simulink model "L22B3"  (R2015a)
settings: Solver=ode45  StartTime=0.0  StopTime=1  MaxStep=0.001  RelTol=1e-3
values from neighbouring files (symbols this model uses):
  bB3 = 1138537    [L22m.m]
  c = 10000    [L22m.m]
  fi1 = -294.11    [L22m.m]
  fi2 = -10740    [L22m.m]
  J = 0.71e-3    (= 0.00071)    [L22m.m]
  kB3 = 5*1e+7    (= 50000000)    [L22m.m]
  ke = 0.33    [L22m.m]
  km = ke    (= 0.33)    [L22m.m]
  kp = 35    [L22m.m]
  La = 14.28e-3    (= 0.01428)    [L22m.m]
  Ra = 4.2    [L22m.m]
  v = -12    [L22m.m]
  vTime = 0.6    [L22m.m]
  w = 20    [L22m.m]
settings Model: Creator=B014-5  LastModifiedBy=B014-5

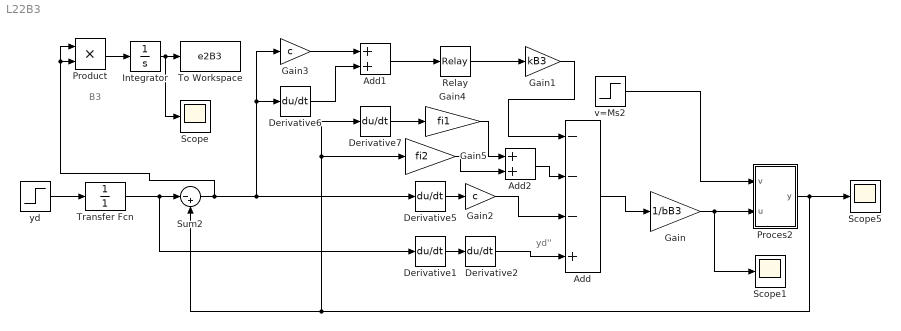
== system L22B3 ==
  note: yd''
  note: B3
  Add : Sum  Inputs=---+
  Add1 : Sum
  Add2 : Sum
  Derivative{1..2,5..7} (5 alike) : Derivative  CoefficientInTFapproximation=1e+5
  Gain : Gain  Gain=1/bB3
  Gain1 : Gain  Gain=kB3
  Gain2 : Gain  Gain=c
  Gain3 : Gain  Gain=c
  Gain4 : Gain  Gain=fi1
  Gain5 : Gain  Gain=fi2
  Integrator : Integrator
  Proces2 : Subsystem
  Product : Product
  Relay : Relay  OnSwitchValue=0  OffSwitchValue=0  OffOutputValue=-1  ZeroCross=off
  Scope : Scope
  Scope1 : Scope
      settings: YMin=-4.25e+105  YMax=0
  Scope5 : Scope
      settings: YMin=-4.25e+105  YMax=0  SaveName=ScopeData6
  Sum2 : Sum  Inputs=|-+
  To Workspace : ToWorkspace  VariableName=e2B3  SampleTime=-1
  Transfer Fcn : TransferFcn  Denominator=[0.0 1]
  v=Ms2 : Step  Time=vTime  After=v  SampleTime=0
  yd : Step  Time=0  After=w  SampleTime=0
  wires:
  Derivative1/1 -> Derivative2/1
  Proces2/1(y) -> Scope5/1, Sum2/2, Gain5/1, Derivative7/1
  Derivative5/1 -> Gain2/1
  v=Ms2/1 -> Proces2/1(v)
  Add/1 -> Gain/1
  Gain2/1 -> Add/3
  Add1/1 -> Relay/1
  Derivative6/1 -> Add1/2
  Gain3/1 -> Add1/1
  Relay/1 -> Gain1/1
  Gain1/1 -> Add/1
  Derivative7/1 -> Gain4/1
  Gain/1 -> Scope1/1, Proces2/2(u)
  Sum2/1 -> Gain3/1, Derivative6/1, Derivative5/1, Product/1, Product/2
  Product/1 -> Integrator/1
  Integrator/1 -> Scope/1, To Workspace/1
  Derivative2/1 -> Add/4
  Add2/1 -> Add/2
  Gain4/1 -> Add2/1
  Gain5/1 -> Add2/2
  yd/1 -> Transfer Fcn/1
  Transfer Fcn/1 -> Derivative1/1, Sum2/1

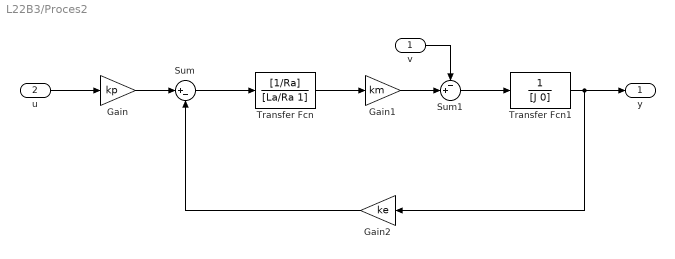
== system L22B3/Proces2 ==
  v : Inport
  u : Inport  Port=2
  Gain : Gain  Gain=kp
  Gain1 : Gain  Gain=km
  Gain2 : Gain  Gain=ke
  Sum : Sum  Inputs=|+-
  Sum1 : Sum  Inputs=-+|
  Transfer Fcn : TransferFcn  Numerator=[1/Ra]  Denominator=[La/Ra 1]
  Transfer Fcn1 : TransferFcn  Denominator=[J 0]
  y : Outport
  wires:
  Transfer Fcn/1 -> Gain1/1
  Gain1/1 -> Sum1/2
  u/1 -> Gain/1
  Gain2/1 -> Sum/2
  Sum/1 -> Transfer Fcn/1
  Sum1/1 -> Transfer Fcn1/1
  Transfer Fcn1/1 -> Gain2/1, y/1
  Gain/1 -> Sum/1
  v/1 -> Sum1/1
